simulink model "PMSM_d_q_sim2"  (R2019a)
settings: Solver=FixedStepAuto  StartTime=0.0  StopTime=500  FixedStep=0.0001  RelTol=1e-3
values from neighbouring files (symbols this model uses):
  f = 0.1    [PMSM_d_q.m]
  Fie = 2.3036    [PMSM_d_q.m]
  J = 0.00529    [PMSM_d_q.m]
  Ld = 0.86431    [PMSM_d_q.m]
  Lq = 0.86431    [PMSM_d_q.m]
  Rs = 0.032988    [PMSM_d_q.m]
  Vs = 1    [PMSM_d_q.m]
settings Model: Creator=TOSHIBA  LastModifiedBy=TOSHIBA

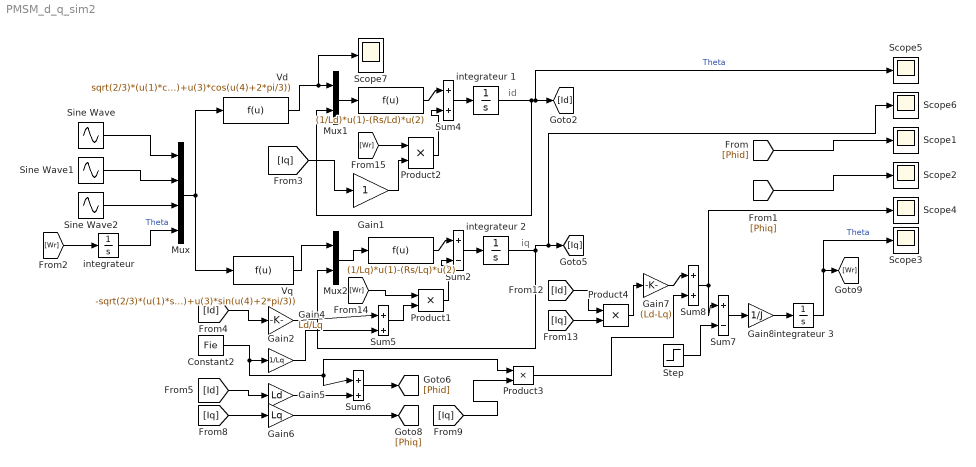
== system PMSM_d_q_sim2 ==
  note: iq
  note: id
  " " : Fcn  Expr=(1/Ld)*u(1)-(Rs/Ld)*u(2)
  " " : Fcn  Expr=(1/Lq)*u(1)-(Rs/Lq)*u(2)
  Constant2 : Constant  Value=Fie
  Gain1 : Gain
  Gain2 : Gain  Gain=1/Lq
  Gain4 : Gain  Gain=Ld/Lq
  Gain5 : Gain  Gain=Ld
  Gain6 : Gain  Gain=Lq
  Gain7 : Gain  Gain=(Ld-Lq)
  Gain8 : Gain  Gain=1/J
  Mux : Mux
  Mux1 : Mux  Inputs=2
  Mux2 : Mux  Inputs=2
  Product{1..4} (4 alike) : Product
  Scope{1..7} (7 alike) : Scope
  Sine Wave : Sin  Amplitude=Vs  Frequency=f*pi*2  SampleTime=0
  Sine Wave1 : Sin  Amplitude=Vs  Frequency=f*pi*2  Phase=-2*pi/3  SampleTime=0
  Sine Wave2 : Sin  Amplitude=Vs  Frequency=f*pi*2  Phase=2*pi/3  SampleTime=0
  Step : Step  Time=0.2  After=0.5  SampleTime=0
  Sum2 : Sum  Inputs=|+-
  Sum{4..6,8} (4 alike) : Sum  Inputs=|++
  Sum7 : Sum  Inputs=|+-
  Vd : Fcn  Expr=sqrt(2/3)*(u(1)*cos(u(4))+u(2)*cos(u(4)-2*pi/3)+u(3)*cos(u(4)+2*pi/3))
  Vq : Fcn  Expr=-sqrt(2/3)*(u(1)*sin(u(4))+u(2)*sin(u(4)-2*pi/3)+u(3)*sin(u(4)+2*pi/3))
  integrateur {,1..3} (4 alike) : Integrator
  wires:
  Sine Wave/1 -> Mux/1
  Sine Wave2/1 -> Mux/3
  [Wr] -> "integrateur "/1
  Mux/1 -> Vq/1, Vd/1
  Sine Wave1/1 -> Mux/2
  "integrateur "/1 -> Mux/4  "Theta"
  Mux1/1 -> " "/1
  " "/1 -> Sum4/1
  Product2/1 -> Sum4/2
  [Wr] -> Product2/1
  Gain1/1 -> Product2/2
  Mux2/1 -> " "/1
  Product1/1 -> Sum2/2
  Sum5/1 -> Product1/2
  " "/1 -> Sum2/1
  Sum2/1 -> integrateur 2/1
  [Wr] -> Product1/1
  Gain4/1 -> Sum5/1
  Gain2/1 -> Sum5/2
  Sum4/1 -> integrateur 1/1
  integrateur 1/1 -> Mux1/2, Scope5/1, [Id]  "Theta"
  integrateur 2/1 -> Scope6/1, [Iq], Mux2/2
  [Iq] -> Gain1/1
  [Id] -> Gain4/1
  [Id] -> Gain5/1
  Constant2/1 -> Gain2/1, Product3/1, Sum6/1
  [Iq] -> Gain6/1
  Gain6/1 -> [Phiq]
  [Iq] -> Product3/2
  [Id] -> Product4/1
  [Iq] -> Product4/2
  Product4/1 -> Gain7/1
  Gain7/1 -> Sum8/1
  Product3/1 -> Sum8/2
  Step/1 -> Sum7/2
  Sum7/1 -> Gain8/1
  Sum8/1 -> Sum7/1, Scope4/1
  Gain8/1 -> integrateur 3/1
  integrateur 3/1 -> Scope3/1, [Wr]  "Theta"
  [Phid] -> Scope1/1
  [Phiq] -> Scope2/1
  Vd/1 -> Scope7/1, Mux1/1
  Vq/1 -> Mux2/1
  Gain5/1 -> Sum6/2
  Sum6/1 -> [Phid]
